simulink model "simulate_PI_controller"  (R2024b)
settings: Solver=ode4  StartTime=0.0  StopTime=Tfin  FixedStep=Tc  RelTol=1e-3
undefined symbols (not defined in the file): Kp_2, Ti_2
settings Model: Creator=martinhaugen  LastModifiedBy=martinhaugen

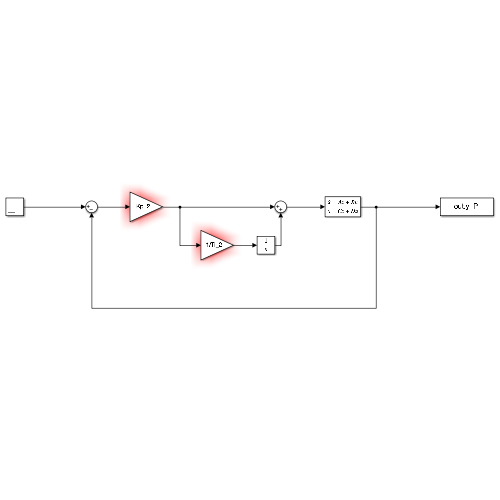
[thumbnail: Simulink's stored preview of the top-level diagram]
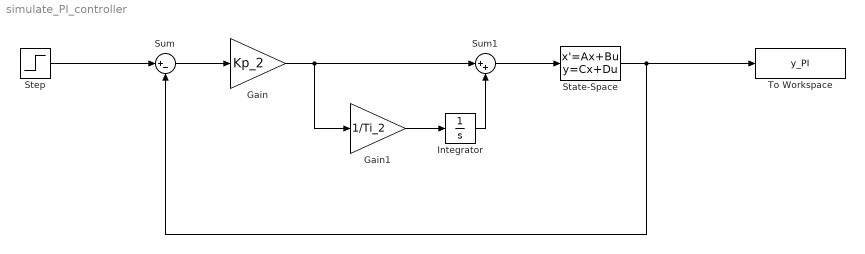
== system simulate_PI_controller ==
  Gain : Gain  Gain=Kp_2
  Gain1 : Gain  Gain=1/Ti_2
  Integrator : Integrator
  State-Space : StateSpace  InitialCondition=0
  Step : Step  Time=0  SampleTime=0
  Sum : Sum  Inputs=|+-
  Sum1 : Sum  Inputs=|++
  To Workspace : ToWorkspace  VariableName=y_PI  SampleTime=-1
  wires:
  Step/1 -> Sum/1
  Sum/1 -> Gain/1
  State-Space/1 -> To Workspace/1, Sum/2
  Sum1/1 -> State-Space/1
  Integrator/1 -> Sum1/2
  Gain/1 -> Sum1/1, Gain1/1
  Gain1/1 -> Integrator/1
